simulink model "fmquestion3"  (R2023b)
settings: Solver=VariableStepAuto  StartTime=0.0  StopTime=1  RelTol=1e-3
libraries: commsynccomp2 x2, commchan3 x1, dspfdesign x1
settings Model: Creator=lenovo  LastModifiedBy=waran
settings ModelReferenceCC: EnableRefExpFcnMdlSchedulingChecks=on

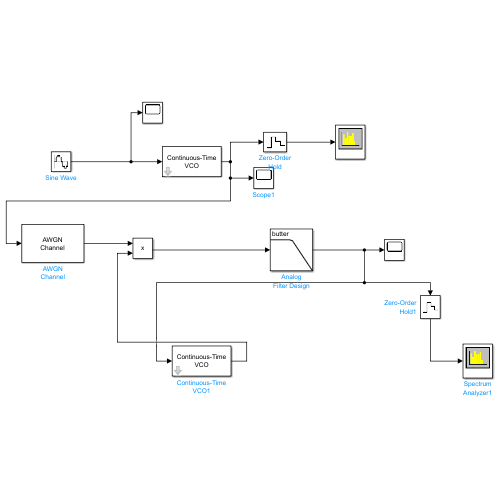
[thumbnail: Simulink's stored preview of the top-level diagram]
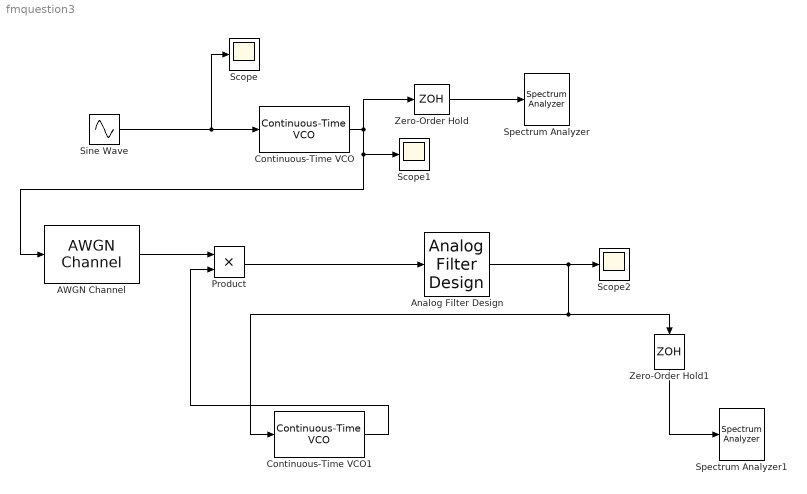
== system fmquestion3 ==
  AWGN Channel : commchan3/AWGN Channel  LegacyMode=on  NoiseMethod="Signal to noise ratio  (SNR)"  noiseMode=Variance from mask  EbNo=10  EsNo=10  SNR=10  BitsPerSymbol=1  SignalPower=1  SamplesPerSymbol=1  SymbolPeriod=1  VarianceSource=Parameter  Variance=0.01  RandomStream=Global stream  Seed=67  SimulateUsing=Code generation
  Analog Filter Design : dspfdesign/Analog Filter Design  method=Butterworth  filttype=Lowpass  N=6  Wlo=2*pi*2000  Whi=80  Rp=2  Rs=40
  Continuous-Time VCO : commsynccomp2/Continuous-Time VCO  Ac=1  Fc=10000  Kc=2500  Ph=0
  Continuous-Time VCO1 : commsynccomp2/Continuous-Time VCO  Ac=1  Fc=10000  Kc=2500  Ph=0
  Product : Product
  Scope : Scope
  Scope1 : Scope
  Scope2 : Scope
  Sine Wave : Sin  Frequency=2*pi*2000  SampleTime=1e-5
  Spectrum Analyzer : SpectrumAnalyzer  WindowPosition=[1.000000,49.000000,1603.000000,779.000000,]  Visible=on  ScopeFrameLocation=window  SampleRateSource=Property  SampleRate=100000  Span=Full  StartFrequency=-50000  StopFrequency=50000  AveragingMethod=Exponential  YLimits=[-102.30428831977381776,32.093024156656930757]
  Spectrum Analyzer1 : SpectrumAnalyzer  WindowPosition=[1 49.4173913043478 1602.78260869565 778.852173913043]  SampleRateSource=Property  SampleRate=100000  StartFrequency=-50000  StopFrequency=50000  AveragingMethod=Exponential  YLimits=[-226.03171510858734905,45.245108379639241036]
  Zero-Order Hold : ZeroOrderHold  SampleTime=1e-5
  Zero-Order Hold1 : ZeroOrderHold  SampleTime=1e-5
  wires:
  Sine Wave/1 -> Scope/1, Continuous-Time VCO/1
  Continuous-Time VCO/1 -> Scope1/1, AWGN Channel/1, Zero-Order Hold/1
  AWGN Channel/1 -> Product/1
  Product/1 -> Analog Filter Design/1
  Analog Filter Design/1 -> Continuous-Time VCO1/1, Zero-Order Hold1/1, Scope2/1
  Continuous-Time VCO1/1 -> Product/2
  Zero-Order Hold1/1 -> Spectrum Analyzer1/1
  Zero-Order Hold/1 -> Spectrum Analyzer/1
